simulink model "pid_position2"  (R2016b)
settings: Solver=ode4  StartTime=0.0  StopTime=20  FixedStep=0.02  RelTol=1e-3
values from neighbouring files (symbols this model uses):
  Kd = -(1/(num(2,3)+num(2,4))*(poles(1)+poles(2)+poles(3))+den(1,2)/(num(2,3)+num(2,4)))*pi/180    [position1.m]    (also in position2.m = (1/(num(2,3)+num(2,4))*(poles(1)+poles(2)+poles(3))+den(1,2))
  Kd_p = 0    [position1.m]    (also in position2.m = 4.87)
  Ki = -(1/(num(2,3)+num(2,4))*(poles(1)*poles(2)*poles(3))+den(1,4)/(num(2,3)+num(2,4)))*pi/180    [position1.m]    (also in position2.m = (1/(num(2,3)+num(2,4))*(poles(1)*poles(2)*poles(3))+den(1,4))
  Ki_p = 0    [position1.m]    (also in position2.m = 0.197)
  Kp = -(den(1,3)/(num(2,3)+num(2,4))-1/(num(2,3)+num(2,4))*(poles(1)*poles(2)+poles(1)*poles(3)+poles(2)*poles(3)))*pi/180    [position1.m]    (also in position2.m = (den(1,3)/(num(2,3)+num(2,4))-1/(num(2,3)+num(2,4))*(poles(1)
  Kp_p = 16.8    [position1.m]    (also in position2.m = 1.96)
  rho = [-1.71136748701 2.88809791639 8.34085809492 -3.97806529373]    [parameters.mat]
  sig = [11.0155519472 -6.53364462652 33.0155389324 0.441275229296 1.60033572418]    [parameters.mat]
undefined symbols (not defined in the file or in its folder): den, num
settings Model: Creator=Ernie  LastModifiedBy=Ernie

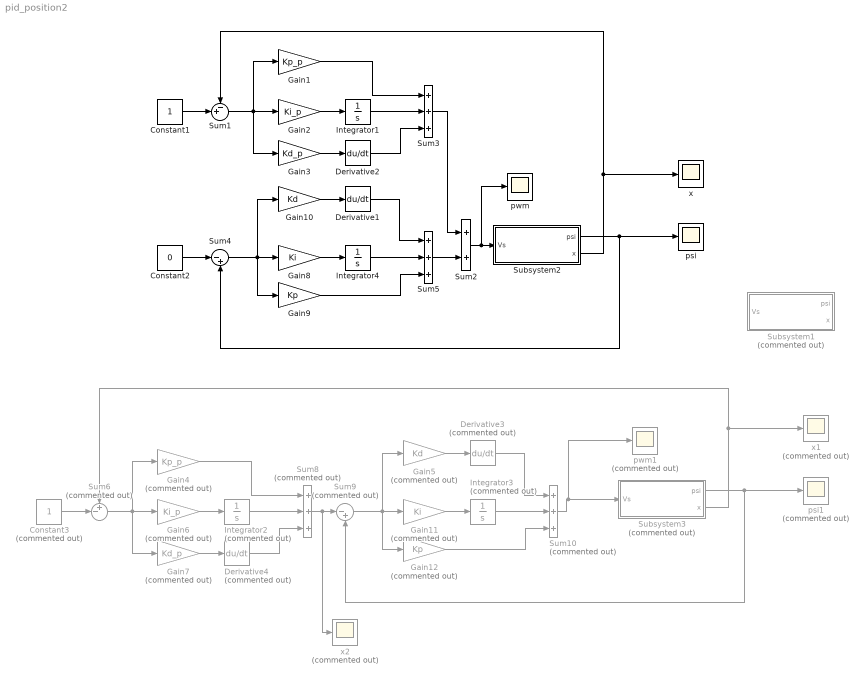
== system pid_position2 ==
  Constant1 : Constant
  Constant2 : Constant  Value=0
  Constant3 : Constant  Commented=on
  Derivative1 : Derivative
  Derivative2 : Derivative
  Derivative3 : Derivative  Commented=on
  Derivative4 : Derivative  Commented=on
  Gain1 : Gain  Gain=Kp_p
  Gain10 : Gain  Gain=Kd
  Gain11 : Gain  Commented=on  Gain=Ki
  Gain12 : Gain  Commented=on  Gain=Kp
  Gain2 : Gain  Gain=Ki_p
  Gain3 : Gain  Gain=Kd_p
  Gain4 : Gain  Commented=on  Gain=Kp_p
  Gain5 : Gain  Commented=on  Gain=Kd
  Gain6 : Gain  Commented=on  Gain=Ki_p
  Gain7 : Gain  Commented=on  Gain=Kd_p
  Gain8 : Gain  Gain=Ki
  Gain9 : Gain  Gain=Kp
  Integrator1 : Integrator
  Integrator2 : Integrator  Commented=on
  Integrator3 : Integrator  Commented=on
  Integrator4 : Integrator
  Subsystem1 : Subsystem  Commented=on
  Subsystem2 : Subsystem
  Subsystem3 : Subsystem  Commented=on
  Sum1 : Sum  Inputs=-+|
  Sum10 : Sum  Commented=on  Inputs=+++
  Sum2 : Sum
  Sum3 : Sum  Inputs=+++
  Sum4 : Sum  Inputs=|-+
  Sum5 : Sum  Inputs=+++
  Sum6 : Sum  Commented=on  Inputs=+-|
  Sum8 : Sum  Commented=on  Inputs=+++
  Sum9 : Sum  Commented=on  Inputs=|-+
  psi : Scope
  psi1 : Scope  Commented=on
  pwm : Scope
  pwm1 : Scope  Commented=on
  x : Scope
  x1 : Scope  Commented=on
  x2 : Scope  Commented=on
  wires:
  Constant2/1 -> Sum4/1
  Gain8/1 -> Integrator4/1
  Integrator4/1 -> Sum5/2
  Gain9/1 -> Sum5/3
  Derivative1/1 -> Sum5/1
  Gain10/1 -> Derivative1/1
  Sum4/1 -> Gain10/1, Gain9/1, Gain8/1
  Subsystem2/1(psi) -> psi/1, Sum4/2
  Constant1/1 -> Sum1/2
  Subsystem2/2(x) -> Sum1/1, x/1
  Sum5/1 -> Sum2/2
  Sum2/1 -> pwm/1, Subsystem2/1(Vs)
  Sum1/1 -> Gain3/1, Gain2/1, Gain1/1
  Gain3/1 -> Derivative2/1
  Gain2/1 -> Integrator1/1
  Sum3/1 -> Sum2/1
  Derivative2/1 -> Sum3/3
  Integrator1/1 -> Sum3/2
  Gain1/1 -> Sum3/1
  Sum8/1 -> x2/1, Sum9/1
  Gain11/1 -> Integrator3/1
  Integrator3/1 -> Sum10/2
  Gain12/1 -> Sum10/3
  Derivative3/1 -> Sum10/1
  Gain5/1 -> Derivative3/1
  Sum9/1 -> Gain5/1, Gain12/1, Gain11/1
  Subsystem3/1(psi) -> psi1/1, Sum9/2
  Constant3/1 -> Sum6/2
  Subsystem3/2(x) -> Sum6/1, x1/1
  Sum6/1 -> Gain7/1, Gain6/1, Gain4/1
  Gain7/1 -> Derivative4/1
  Gain6/1 -> Integrator2/1
  Derivative4/1 -> Sum8/3
  Integrator2/1 -> Sum8/2
  Gain4/1 -> Sum8/1
  Sum10/1 -> Subsystem3/1(Vs), pwm1/1

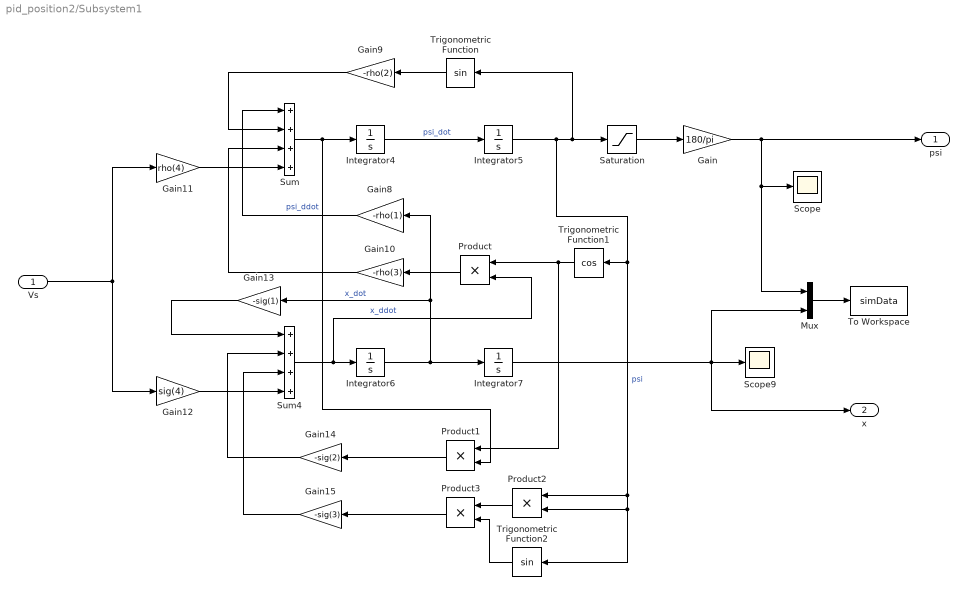
== system pid_position2/Subsystem1 ==
  Vs : Inport
  Gain : Gain  Gain=180/pi
  Gain10 : Gain  Gain=-rho(3)
  Gain11 : Gain  Gain=rho(4)
  Gain12 : Gain  Gain=sig(4)
  Gain13 : Gain  Gain=-sig(1)
  Gain14 : Gain  Gain=-sig(2)
  Gain15 : Gain  Gain=-sig(3)
  Gain8 : Gain  Gain=-rho(1)
  Gain9 : Gain  Gain=-rho(2)
  Integrator4 : Integrator
  Integrator5 : Integrator  InitialCondition=5*pi/180
  Integrator6 : Integrator
  Integrator7 : Integrator
  Mux : Mux  Inputs=2
  Product{,1..3} (4 alike) : Product
  Saturation : Saturate  UpperLimit=pi/2  LowerLimit=-pi/2
  Scope : Scope
  Scope9 : Scope
  Sum : Sum  Inputs=++++
  Sum4 : Sum  Inputs=++++
  To Workspace : ToWorkspace  VariableName=simData  SaveFormat=Timeseries  SampleTime=-1
  Trigonometric Function : Trigonometry
  Trigonometric Function1 : Trigonometry  Operator=cos
  Trigonometric Function2 : Trigonometry
  psi : Outport
  x : Outport  Port=2
  wires:
  Integrator4/1 -> Integrator5/1  "psi_dot"
  Integrator6/1 -> Gain13/1, Gain8/1, Integrator7/1  "x_dot"
  Sum4/1 -> Product/2, Integrator6/1  "x_ddot"
  Sum/1 -> Product1/2, Integrator4/1  "psi_ddot"
  Gain8/1 -> Sum/1
  Trigonometric Function/1 -> Gain9/1
  Integrator5/1 -> Trigonometric Function2/1, Product2/2, Product2/1, Trigonometric Function1/1, Saturation/1, Trigonometric Function/1  "psi"
  Gain9/1 -> Sum/2
  Product/1 -> Gain10/1
  Trigonometric Function1/1 -> Product1/1, Product/1
  Gain10/1 -> Sum/3
  Gain11/1 -> Sum/4
  Gain12/1 -> Sum4/4
  Gain13/1 -> Sum4/1
  Product1/1 -> Gain14/1
  Gain14/1 -> Sum4/2
  Product2/1 -> Product3/1
  Trigonometric Function2/1 -> Product3/2
  Product3/1 -> Gain15/1
  Gain15/1 -> Sum4/3
  Integrator7/1 -> x/1, Mux/2, Scope9/1
  Mux/1 -> To Workspace/1
  Vs/1 -> Gain12/1, Gain11/1
  Gain/1 -> Mux/1, Scope/1, psi/1
  Saturation/1 -> Gain/1

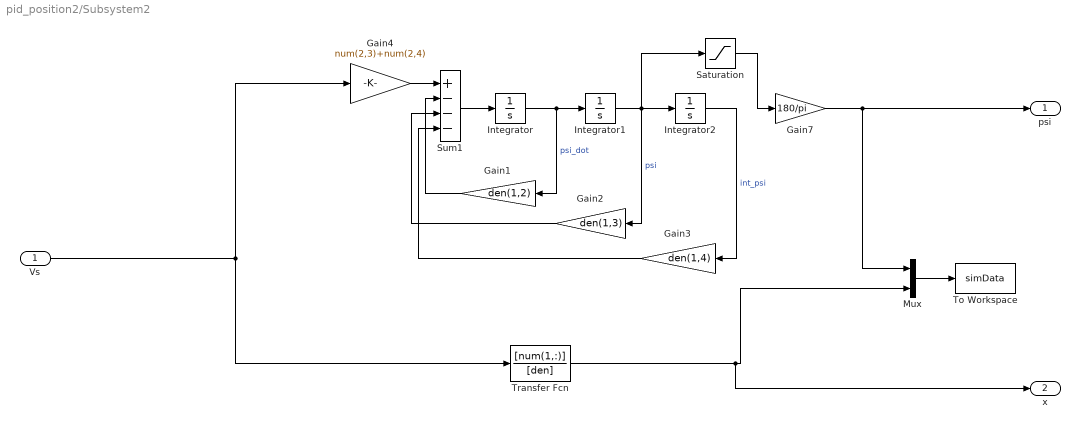
== system pid_position2/Subsystem2 ==
  Vs : Inport
  Gain1 : Gain  Gain=den(1,2)
  Gain2 : Gain  Gain=den(1,3)
  Gain3 : Gain  Gain=den(1,4)
  Gain4 : Gain  Gain=num(2,3)+num(2,4)
  Gain7 : Gain  Gain=180/pi
  Integrator : Integrator
  Integrator1 : Integrator  InitialCondition=10*pi/180
  Integrator2 : Integrator
  Mux : Mux  Inputs=2
  Saturation : Saturate  UpperLimit=pi/2  LowerLimit=-pi/2
  Sum1 : Sum  Inputs=+---
  To Workspace : ToWorkspace  VariableName=simData  SaveFormat=Timeseries  SampleTime=-1
  Transfer Fcn : TransferFcn  Numerator=[num(1,:)]  Denominator=[den]
  psi : Outport
  x : Outport  Port=2
  wires:
  Mux/1 -> To Workspace/1
  Gain7/1 -> Mux/1, psi/1
  Integrator/1 -> Gain1/1, Integrator1/1  "psi_dot"
  Integrator1/1 -> Saturation/1, Gain2/1, Integrator2/1  "psi"
  Sum1/1 -> Integrator/1
  Gain1/1 -> Sum1/2
  Gain2/1 -> Sum1/3
  Integrator2/1 -> Gain3/1  "int_psi"
  Gain3/1 -> Sum1/4
  Gain4/1 -> Sum1/1
  Saturation/1 -> Gain7/1
  Transfer Fcn/1 -> x/1, Mux/2
  Vs/1 -> Transfer Fcn/1, Gain4/1

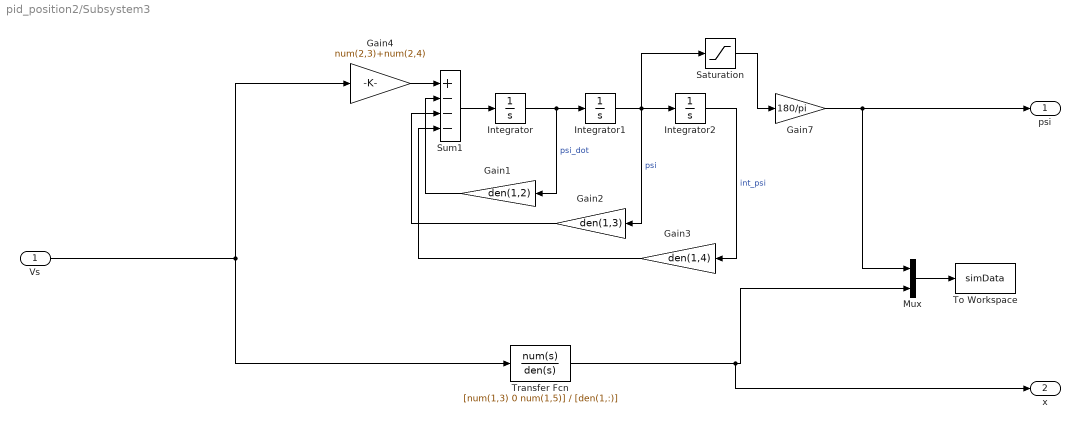
== system pid_position2/Subsystem3 ==
  Vs : Inport
  Gain1 : Gain  Gain=den(1,2)
  Gain2 : Gain  Gain=den(1,3)
  Gain3 : Gain  Gain=den(1,4)
  Gain4 : Gain  Gain=num(2,3)+num(2,4)
  Gain7 : Gain  Gain=180/pi
  Integrator : Integrator
  Integrator1 : Integrator  InitialCondition=0*pi/180
  Integrator2 : Integrator
  Mux : Mux  Inputs=2
  Saturation : Saturate  UpperLimit=pi/2  LowerLimit=-pi/2
  Sum1 : Sum  Inputs=+---
  To Workspace : ToWorkspace  VariableName=simData  SaveFormat=Timeseries  SampleTime=-1
  Transfer Fcn : TransferFcn  Numerator=[num(1,3) 0 num(1,5)]  Denominator=[den(1,:)]
  psi : Outport
  x : Outport  Port=2
  wires:
  Mux/1 -> To Workspace/1
  Gain7/1 -> Mux/1, psi/1
  Integrator/1 -> Gain1/1, Integrator1/1  "psi_dot"
  Integrator1/1 -> Saturation/1, Gain2/1, Integrator2/1  "psi"
  Sum1/1 -> Integrator/1
  Gain1/1 -> Sum1/2
  Gain2/1 -> Sum1/3
  Integrator2/1 -> Gain3/1  "int_psi"
  Gain3/1 -> Sum1/4
  Gain4/1 -> Sum1/1
  Saturation/1 -> Gain7/1
  Transfer Fcn/1 -> x/1, Mux/2
  Vs/1 -> Transfer Fcn/1, Gain4/1
